simulink model "MPC_bias"  (R2018b)
settings: Solver=VariableStepAuto  StartTime=0.0  StopTime=5  RelTol=1e-3
undefined symbols (not defined in the file or in its folder): Discrete, Time
libraries: ctrlSharedLib x1, mpclib x1
settings Model: Creator=dongdaming  LastModifiedBy=dongdaming

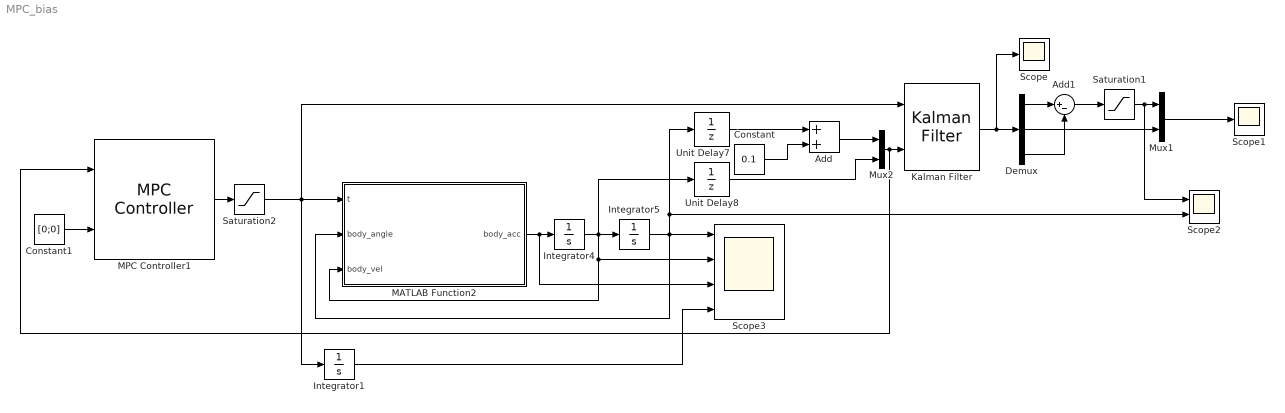
== system MPC_bias ==
  Add : Sum
  Add1 : Sum  Inputs=|+-
  Constant : Constant  Value=0.1
  Constant1 : Constant  Value=[0;0]
  Demux : Demux  Outputs=3
  Integrator1 : Integrator
  Integrator4 : Integrator
  Integrator5 : Integrator  InitialCondition=pi/3  UpperSaturationLimit=pi  LowerSaturationLimit=-pi
  Kalman Filter : ctrlSharedLib/Kalman Filter  TimeDomain=Discrete-Time  UseCurrentEstimator=on  ModelSource=Individual A, B, C, D matrices  ModelSourceVariable=ss(0.95,1,1,0,1)  A=[0,1,-1;3.649100000000000e+02,0,0;0,0,1]  B=[0;-8.422600000000000e+02;0]  C=[1 0 0;0 1 0]  D=[0;0]  NumberOfStates=1  NumberOfInputs=1  NumberOfOutputs=1  InitialEstimateSource=Dialog  X0=[pi/3;0;0]  P0=10  UseK=off  UseGH=off  NumberOfProcessNoiseInputs=1  G=1  TimeInvariantG=on  H=0  TimeInvariantH=on  Q=[0.1 0 0;0 0.1 0; 0 0 0.1]  TimeInvariantQ=on  R=[1 0 ; 0 1 ]  TimeInvariantR=on  N=0  TimeInvariantN=on  AddInputPort=on  AddEnablePort=off  OutputEstimatedY=off  OutputP=off  Ts=-1
      settings: SourceProductBaseCode=CT
  MATLAB Function2 : MATLAB Function  TreatAsAtomicUnit=on
  MPC Controller1 : mpclib/MPC Controller  SCDEnableBlockLinearizationSpecification=on  mpcobj=mpc1  is_multiple=0  enable_value=0  return_u0=off  updateMPCinCallerWorkspace=on  md_inport=off  mv_inport=off  return_cost=off  return_mvseq=off  return_qpstatus=off  return_xseq=off  return_state=off  return_ovseq=off  state_inport=off  umin_inport=off  umax_inport=off  ymin_inport=off  ymax_inport=off  cc_inport=off  ywt_inport=off  uwt_inport=off  duwt_inport=off  rhoeps_inport=off  uref_inport=off  n_ts=0.002  n_p=20  n_mv=1  n_md=0  n_ud=0  n_mo=2  n_uo=0  BlockDataType=double  SampleTimeInherited=off  switch_inport=off
  Mux1 : Mux  Inputs=2
  Mux2 : Mux  Inputs=2
  Saturation1 : Saturate  UpperLimit=pi/2  LowerLimit=-pi/2
  Saturation2 : Saturate  UpperLimit=1.4  LowerLimit=-1.4
  Scope : Scope
  Scope1 : Scope
  Scope2 : Scope  NumInputPorts=2
  Scope3 : Scope  NumInputPorts=4
  Unit Delay7 : UnitDelay  SampleTime=0.002
  Unit Delay8 : UnitDelay  InitialCondition=pi/3  SampleTime=0.002
  wires:
  Unit Delay8/1 -> Mux2/2
  MPC Controller1/1 -> Saturation2/1
  Saturation2/1 -> MATLAB Function2/1(t), Kalman Filter/1, Integrator1/1
  MATLAB Function2/1(body_acc) -> Integrator4/1, Scope3/3
  Mux2/1 -> MPC Controller1/1, Kalman Filter/2
  Constant1/1 -> MPC Controller1/2
  Integrator5/1 -> Scope3/1, MATLAB Function2/2(body_angle), Scope2/2, Unit Delay7/1
  Integrator4/1 -> Integrator5/1, Scope3/2, MATLAB Function2/3(body_vel), Unit Delay8/1
  Unit Delay7/1 -> Add/1
  Add/1 -> Mux2/1
  Constant/1 -> Add/2
  Integrator1/1 -> Scope3/4
  Kalman Filter/1 -> Scope/1, Demux/1
  Demux/1 -> Add1/1
  Demux/3 -> Add1/2
  Add1/1 -> Saturation1/1
  Demux/2 -> Mux1/2
  Mux1/1 -> Scope1/1
  Saturation1/1 -> Scope2/1, Mux1/1

== matlab function MPC_bias/MATLAB Function2 ==
  data: t input; body_acc output; body_angle input; body_vel input
function body_acc = fcn(t,body_angle,body_vel)
body_acc=(+1429.48*sin(body_angle)-1215.55*t-2083.85*t*cos(body_angle)-3.87597*sin(2*body_angle)*body_vel^2)/(2.91931+cos(body_angle)^2+8.75194*sin(body_angle)^2);
